simulink model "prelab"  (R2015b)
settings: Solver=VariableStepAuto  StartTime=0.0  StopTime=4  MaxStep=0.01  RelTol=1e-3
settings Model: Creator=WangRui  LastModifiedBy=WangRui
settings SolverCC: ZeroCrossControl=DisableAll
settings DataIOCC: LimitDataPoints=off

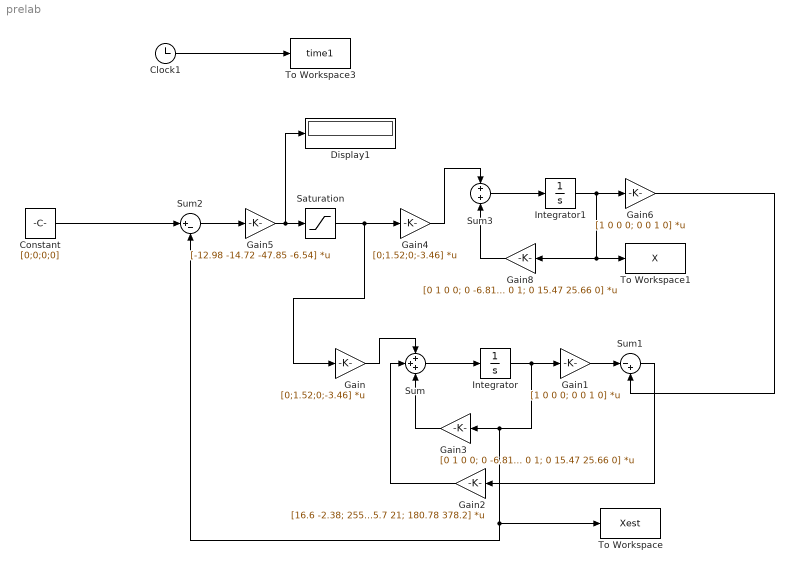
== system prelab ==
  Clock1 : Clock
  Constant : Constant  Value=[0;0;0;0]
  Display1 : Display
  Gain : Gain  Gain=[0;1.52;0;-3.46]  Multiplication=Matrix(K*u)
  Gain1 : Gain  Gain=[1 0 0 0; 0 0 1 0]  Multiplication=Matrix(K*u)
  Gain2 : Gain  Gain=[16.6 -2.38; 255 -5.49; 15.7 21; 180.78 378.2]  Multiplication=Matrix(K*u)
  Gain3 : Gain  Gain=[0 1 0 0; 0 -6.81 -1.5 0; 0 0 0 1; 0 15.47 25.66 0]  Multiplication=Matrix(K*u)
  Gain4 : Gain  Gain=[0;1.52;0;-3.46]  Multiplication=Matrix(K*u)
  Gain5 : Gain  Gain=[-12.98 -14.72 -47.85 -6.54]  Multiplication=Matrix(K*u)
  Gain6 : Gain  Gain=[1 0 0 0; 0 0 1 0]  Multiplication=Matrix(K*u)
  Gain8 : Gain  Gain=[0 1 0 0; 0 -6.81 -1.5 0; 0 0 0 1; 0 15.47 25.66 0]  Multiplication=Matrix(K*u)
  Integrator : Integrator
  Integrator1 : Integrator  InitialCondition=[0.1 0 0.087266 0]
  Saturation : Saturate  UpperLimit=6  LowerLimit=-6
  Sum : Sum  Inputs=+++
  Sum1 : Sum  Inputs=|-+
  Sum2 : Sum  Inputs=|+-
  Sum3 : Sum
  To Workspace : ToWorkspace  VariableName=Xest  SampleTime=-1
      settings: Save2DSignal=2-D array (concatenate along first dimension)
  To Workspace1 : ToWorkspace  VariableName=X  SampleTime=-1
      settings: Save2DSignal=2-D array (concatenate along first dimension)
  To Workspace3 : ToWorkspace  VariableName=time1  SampleTime=-1
  wires:
  Gain/1 -> Sum/1
  Gain2/1 -> Sum/2
  Sum/1 -> Integrator/1
  Integrator/1 -> Gain3/1, To Workspace/1, Sum2/2, Gain1/1
  Gain1/1 -> Sum1/1
  Gain6/1 -> Sum1/2
  Sum1/1 -> Gain2/1
  Gain3/1 -> Sum/3
  Clock1/1 -> To Workspace3/1
  Sum2/1 -> Gain5/1
  Saturation/1 -> Gain/1, Gain4/1
  Gain5/1 -> Display1/1, Saturation/1
  Constant/1 -> Sum2/1
  Gain4/1 -> Sum3/1
  Sum3/1 -> Integrator1/1
  Integrator1/1 -> To Workspace1/1, Gain8/1, Gain6/1
  Gain8/1 -> Sum3/2
